simulink model "SystemsSimulinkQuizBlock"  (R2015a)
settings: Solver=ode45  StartTime=0.0  StopTime=10.0  RelTol=1e-3
values from neighbouring files (symbols this model uses):
  c = 50    [SystemsSimulinkQuiz.m]
  k1 = 2000    [SystemsSimulinkQuiz.m]
  k2 = 2000    [SystemsSimulinkQuiz.m]
  m1 = 500    [SystemsSimulinkQuiz.m]
  m2 = 500    [SystemsSimulinkQuiz.m]
settings Model: Creator=jack  LastModifiedBy=jack

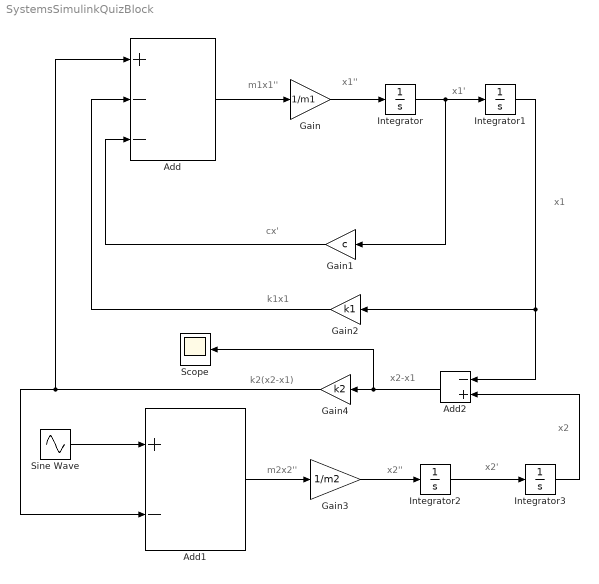
== system SystemsSimulinkQuizBlock ==
  note: k2(x2-x1)
  note: x2-x1
  note: x2
  note: x2'
  note: x2''
  note: m2x2''
  note: x1
  note: k1x1
  note: cx'
  note: x1'
  note: x1''
  note: m1x1''
  Add : Sum  Inputs=+--
  Add1 : Sum  Inputs=+-
  Add2 : Sum  Inputs=-+
  Gain : Gain  Gain=1/m1
  Gain1 : Gain  Gain=c
  Gain2 : Gain  Gain=k1
  Gain3 : Gain  Gain=1/m2
  Gain4 : Gain  Gain=k2
  Integrator{,1..3} (4 alike) : Integrator
  Scope : Scope
      settings: YMin=-1  YMax=1
  Sine Wave : Sin  Amplitude=10  Frequency=2  SampleTime=0
  wires:
  Add/1 -> Gain/1
  Gain/1 -> Integrator/1
  Integrator/1 -> Gain1/1, Integrator1/1
  Gain1/1 -> Add/3
  Integrator1/1 -> Add2/1, Gain2/1
  Gain2/1 -> Add/2
  Sine Wave/1 -> Add1/1
  Add1/1 -> Gain3/1
  Gain3/1 -> Integrator2/1
  Integrator2/1 -> Integrator3/1
  Integrator3/1 -> Add2/2
  Add2/1 -> Scope/1, Gain4/1
  Gain4/1 -> Add/1, Add1/2
